simulink model "s_deng_rev1_13_wide"  (R2016b)
(part 4 of 68)

  Gateway Out93/1 -> To Workspace87/1
  Gateway Out94/1 -> To Workspace88/1
  Gateway Out95/1 -> To Workspace89/1
  Gateway Out96/1 -> To Workspace90/1
  Gateway Out97/1 -> To Workspace91/1
  Gateway Out98/1 -> To Workspace92/1
  Gateway Out99/1 -> To Workspace93/1
  Gateway Out100/1 -> To Workspace94/1
  Constant10/1 -> Terminator/1
  Constant12/1 -> Terminator32/1
  Constant13/1 -> Terminator33/1
  Constant14/1 -> Terminator34/1
  Constant98/1 -> gbe_iptx3/1(sim_1)
  Constant84/1 -> gbe_iptx2/1(sim_1)
  Constant83/1 -> gbe_iptx1/1(sim_1)
  Constant78/1 -> gbe_iptx0/1(sim_1)
  64_to_3/2 -> Mux17/3, bram_munge3/1(In1)
  64_to_1/2 -> Mux16/3, bram_munge2/1(In1)
  64_to_2/2 -> Mux18/3, bram_munge1/1(In1)
  pipeline74/1(q) -> pipeline75/1(d), edge_detect17/1(in)
  64_to_256/2 -> Mux19/3, bram_munge0/1(In1)
  Gateway Out102/1 -> To Workspace96/1
  Concat11/1 -> pipeline164/1(d)
  pipeline164/1(q) -> pipeline168/1(d)
  [sp256_dv1] -> edge_detect15/1(in), Concat11/2
  Constant104/1 -> Mux4/2
  [gbe_ip1] -> Mux4/3
  Concat12/1 -> pipeline69/1(d)
  pipeline69/1(q) -> pipeline153/1(d)
  [gbe_ip0] -> Mux24/3
  Constant103/1 -> Mux24/2
  Gateway Out103/1 -> To Workspace97/1
  [sp256_dv2] -> edge_detect16/1(in), Concat12/1
  [sp256_dv0] -> edge_detect28/1(in), Concat12/2
  [gbe_ip2] -> Mux24/4
  Constant105/1 -> Mux24/5
  [gbe_ip3] -> Mux4/4
  Constant102/1 -> Mux4/5
  pipeline153/1(q) -> pipeline174/1(d), Gateway Out103/1, Mux24/1
  Gateway Out105/1 -> To Workspace99/1
  Concat13/1 -> Gateway Out106/1, Mux27/1
  Slice5/1 -> Logical51/1
  Slice6/1 -> Logical51/2
  Slice7/1 -> Logical52/1
  Slice8/1 -> Logical52/2
  Constant114/1 -> Mux27/2
  Constant128/1 -> Mux27/5
  Logical51/1 -> Concat13/2
  Logical52/1 -> Concat13/1
  Mux4/1 -> Gateway Out128/1, Register/1
  pipeline173/1(q) -> Slice6/1, Slice5/1
  pipeline174/1(q) -> Slice8/1, Slice7/1
  Gateway Out101/1 -> To Workspace95/1
  Gateway Out104/1 -> To Workspace98/1
  Gateway Out106/1 -> To Workspace100/1
  [gbe_ip0] -> Relational15/2
  [gbe_ip1] -> Relational16/2
  [gbe_ip2] -> Relational17/2
  [gbe_ip3] -> Relational18/2
  [msync] -> Counter12/1, Counter11/1, Counter10/1, Counter9/1, Gateway Out111/1
  ip_count0/1(sim_out) -> To Workspace101/1
  Counter9/1 -> ip_count0/1(out_ip_count0)
  Counter12/1 -> ip_count3/1(out_ip_count3)
  Gateway Out111/1 -> To Workspace105/1
  Gateway Out112/1 -> To Workspace106/1
  Gateway Out114/1 -> To Workspace108/1
  Gateway Out115/1 -> To Workspace109/1
  Gateway Out116/1 -> To Workspace110/1
  Counter11/1 -> ip_count2/1(out_ip_count2)
  Counter10/1 -> ip_count1/1(out_ip_count1)
  ip_count1/1(sim_out) -> To Workspace103/1
  ip_count2/1(sim_out) -> To Workspace104/1
  ip_count3/1(sim_out) -> To Workspace107/1
  Relational15/1 -> Gateway Out117/1, Logical53/1
  Relational16/1 -> Gateway Out120/1, Logical54/1
  Logical53/1 -> Gateway Out112/1, Counter9/2
  Logical54/1 -> Counter10/2, Gateway Out114/1
  Logical55/1 -> Counter11/2, Gateway Out115/1
  Relational18/1 -> Gateway Out124/1, Logical56/1
  Logical56/1 -> Counter12/2, Gateway Out116/1
  master_reset_sim10/1 -> ramp_control/1(sim_1)
  master_reset_sim11/1 -> ramp_control/2(sim_2)
  master_reset_sim12/1 -> ramp_control/3(sim_3)
  master_reset_sim13/1 -> ramp_control/4(sim_4)
  Gateway Out107/1 -> To Workspace102/1
  Gateway Out108/1 -> To Workspace111/1
  Gateway Out109/1 -> To Workspace112/1
  Gateway Out110/1 -> To Workspace113/1
  Mux21/1 -> Gateway Out110/1, spead_pack3/3(data64)
  Gateway Out113/1 -> To Workspace114/1
  pipeline168/1(q) -> Gateway Out102/1, Mux4/1, pipeline173/1(d)
  [sp256_eofg1] -> Logical10/2
  [sp256_eofg3] -> Logical10/4
  [gbe_txip] -> Relational18/1, Relational17/1, Relational16/1, Relational15/1
  [sp256_eofg0] -> pipeline183/1(d)
  pipeline183/1(q) -> Gateway Out118/1, Logical53/2
  [sp256_eofg1] -> pipeline184/1(d)
  [sp256_eofg2] -> pipeline185/1(d)
  [sp256_eofg3] -> pipeline192/1(d)
  pipeline184/1(q) -> Gateway Out119/1, Logical54/2
  pipeline185/1(q) -> Gateway Out121/1, Logical55/2
  pipeline192/1(q) -> Gateway Out123/1, Logical56/2
  Gateway Out117/1 -> To Workspace115/1
  Gateway Out118/1 -> To Workspace116/1
  Gateway Out119/1 -> To Workspace117/1
  Gateway Out120/1 -> To Workspace118/1
  Gateway Out121/1 -> To Workspace119/1
  Gateway Out122/1 -> To Workspace120/1
  Relational17/1 -> Gateway Out122/1, Logical55/1
  Gateway Out123/1 -> To Workspace121/1
  Gateway Out124/1 -> To Workspace122/1
  [sp256_dv3] -> edge_detect14/1(in), Concat11/1
  edge_detect14/1(out) -> Logical57/1
  edge_detect15/1(out) -> Logical57/2
  Logical57/1 -> Delay91/1
  Register/1 -> Mux27/3, Gateway Out104/1
  Mux24/1 -> Gateway Out126/1, Register4/1
  Register4/1 -> Gateway Out101/1, Mux27/4
  edge_detect16/1(out) -> Logical58/1
  edge_detect28/1(out) -> Logical58/2
  Logical58/1 -> Delay88/1
  Gateway Out125/1 -> To Workspace123/1
  Gateway Out126/1 -> To Workspace124/1
  Gateway Out127/1 -> To Workspace125/1
  Gateway Out128/1 -> To Workspace126/1
  Delay87/1 -> Gateway Out125/1, Register4/2
  Delay88/1 -> Delay89/1
  Delay89/1 -> Delay87/1
  Delay90/1 -> Gateway Out127/1, Register/2
  Delay91/1 -> Delay92/1
  Delay92/1 -> Delay90/1
  Mux27/1 -> Gateway Out129/1, Register7/1
  Register7/1 -> Gateway Out105/1, [gbe_txip]
  edge_detect30/1(out) -> Logical59/1
  edge_detect31/1(out) -> Logical59/2
  Logical59/1 -> Register7/2, Gateway Out130/1
  Gateway Out129/1 -> To Workspace127/1
  Gateway Out130/1 -> To Workspace128/1
  edge_detect32/1(out) -> Logical59/4
  edge_detect29/1(out) -> Logical59/3
  [sp256_dv0] -> Delay96/1
  [sp256_dv2] -> Delay95/1
  [sp256_dv1] -> Delay94/1
  [sp256_dv3] -> Delay93/1
  Delay93/1 -> edge_detect30/1(in)
  Delay94/1 -> edge_detect31/1(in)
  Delay95/1 -> edge_detect29/1(in)
  Delay96/1 -> edge_detect32/1(in)
  pipeline169/1(q) -> Gateway Out9/1, [sp256_dv]
  pipeline175/1(q) -> Gateway Out12/1, [sp256_eof]
  pipeline193/1(q) -> bus_expand1/1(bus_in), [sp256_data]
  [sp256_dv] -> pipeline226/1(d), edge_detect33/1, pipeline208/1(d)
  [gbe_txip] -> pipeline194/1(d)
  [sp256_eof] -> pipeline196/1(d)
  pipeline194/1(q) -> ss_ip_tx/1(in_ip)
  pipeline196/1(q) -> ss_ip_tx/2(in_eof)
  pipeline208/1(q) -> ss_ip_tx/3(in_dv)
  pipeline226/1(q) -> ss_ip_tx/4(we)
  pipeline230/1(q) -> ss_ip_tx/5(trig)
  edge_detect33/1 -> pipeline230/1(d)
